simulink model "bai2"  (R2017b)
settings: Solver=ode4  StartTime=0.0  StopTime=20  FixedStep=0.01  RelTol=1e-3
libraries: fuzblock x1
settings Model: Creator=phamt  LastModifiedBy=phamt

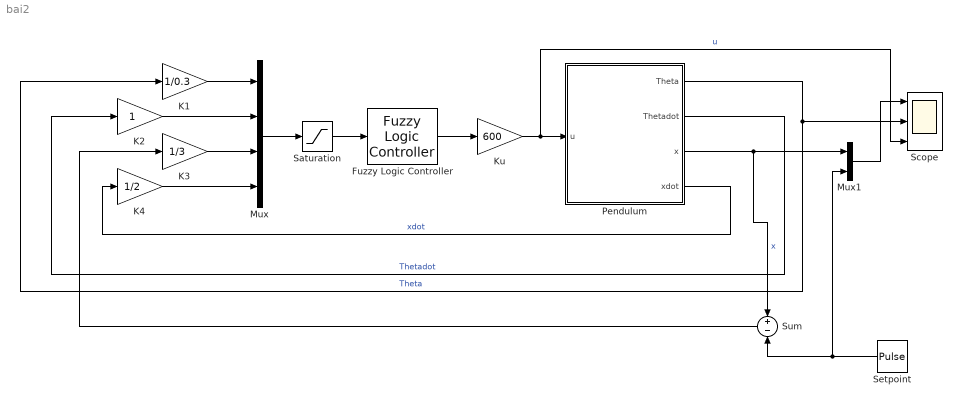
== system bai2 ==
  Fuzzy Logic Controller : fuzblock/Fuzzy Logic  Controller  FIS='bai2_FIS.fis'  OutputSampleNumber=101  DataType=double  FuzzifiedInputs=off  RuleFiringStrengths=off  RuleOutputs=off  AggregatedOutputs=off  SimulateUsing=Interpreted execution
  K1 : Gain  Gain=1/0.3
  K2 : Gain
  K3 : Gain  Gain=1/3
  K4 : Gain  Gain=1/2
  Ku : Gain  Gain=600
  Mux : Mux
  Mux1 : Mux  Inputs=2
  Pendulum : Subsystem  mask{H=5, m=3, l=1, g=9.81, x0=1, xdot0=-1, Theta0=-0.2, Thetadot0=-0.2}
      mask prompts: H "M"
  Saturation : Saturate  UpperLimit=1  LowerLimit=-1
  Scope : Scope  NumInputPorts=3
  Setpoint : DiscretePulseGenerator  PulseType=Time based  Period=20  PulseWidth=50
  Sum : Sum  Inputs=+-
  wires:
  Fuzzy Logic Controller/1 -> Ku/1
  K1/1 -> Mux/1
  Mux/1 -> Saturation/1
  K2/1 -> Mux/2
  Saturation/1 -> Fuzzy Logic Controller/1
  Ku/1 -> Scope/3, Pendulum/1(u)  "u"
  K3/1 -> Mux/3
  K4/1 -> Mux/4
  Pendulum/4(xdot) -> K4/1  "xdot"
  Pendulum/3(x) -> Sum/1, Mux1/1  "x"
  Pendulum/2(Thetadot) -> K2/1  "Thetadot"
  Pendulum/1(Theta) -> Scope/2, K1/1  "Theta"
  Mux1/1 -> Scope/1
  Setpoint/1 -> Mux1/2, Sum/2
  Sum/1 -> K3/1

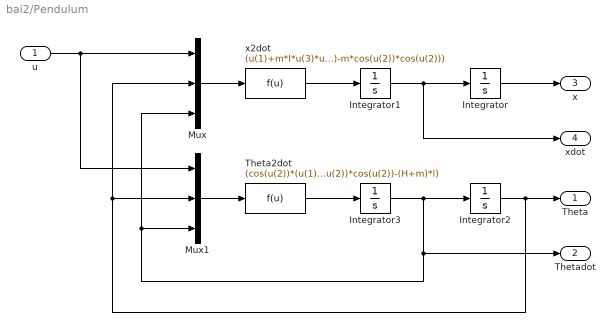
== system bai2/Pendulum ==
  u : Inport
  Integrator : Integrator  InitialCondition=x0
  Integrator1 : Integrator  InitialCondition=xdot0
  Integrator2 : Integrator  InitialCondition=Theta0
  Integrator3 : Integrator  InitialCondition=Thetadot0
  Mux : Mux  Inputs=3
  Mux1 : Mux  Inputs=3
  Theta2dot : Fcn  Expr=(cos(u(2))*(u(1)+m*l*u(3)*u(3)*sin(u(1)))-(H+m)*(g*sin(u(2))))/(m*l*cos(u(2))*cos(u(2))-(H+m)*l)
  x2dot : Fcn  Expr=(u(1)+m*l*u(3)*u(3)*sin(u(2))-m*g*sin(u(2))*cos(u(2)))/((H+m)-m*cos(u(2))*cos(u(2)))
  Theta : Outport
  Thetadot : Outport  Port=2
  x : Outport  Port=3
  xdot : Outport  Port=4
  wires:
  x2dot/1 -> Integrator1/1
  Integrator/1 -> x/1
  Integrator1/1 -> xdot/1, Integrator/1
  Integrator3/1 -> Integrator2/1, Mux/3, Mux1/3, Thetadot/1
  Theta2dot/1 -> Integrator3/1
  u/1 -> Mux/1, Mux1/1
  Integrator2/1 -> Mux/2, Mux1/2, Theta/1
  Mux/1 -> x2dot/1
  Mux1/1 -> Theta2dot/1
